simulink model "SimulinkModelMatlab2022bStudents"  (R2025b)
settings: Solver=VariableStepAuto  StartTime=0.0  StopTime=5e-5  RelTol=1e-3
values from neighbouring files (symbols this model uses):
  Ad = sysDiscreteZOH.A    [pt1.m]
  Bd = sysDiscreteZOH.B    [pt1.m]
  Cd = sysDiscreteZOH.C    [pt1.m]
  Rnsim = 0.0025    [pt1.m]
  Rvsim = [0.025 0; 0 1e-6]    [pt1.m]
  Ts = 2*pi / (10* wn)    [Kalman_code.m]    (also in pt1.m = 2.5e-07)
settings Model: Creator=Freja  LastModifiedBy=Lenovo
settings DataIOCC: ReturnWorkspaceOutputs=off
settings OptimizationCC: ReuseModelBlockBuffer=off
settings RTWCC: GPUComputeCapability=3.5

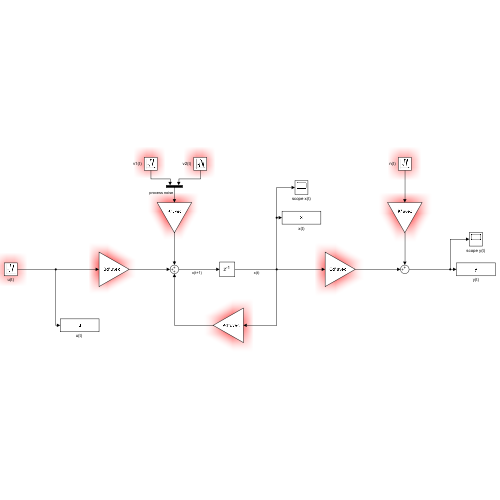
[thumbnail: Simulink's stored preview of the top-level diagram]
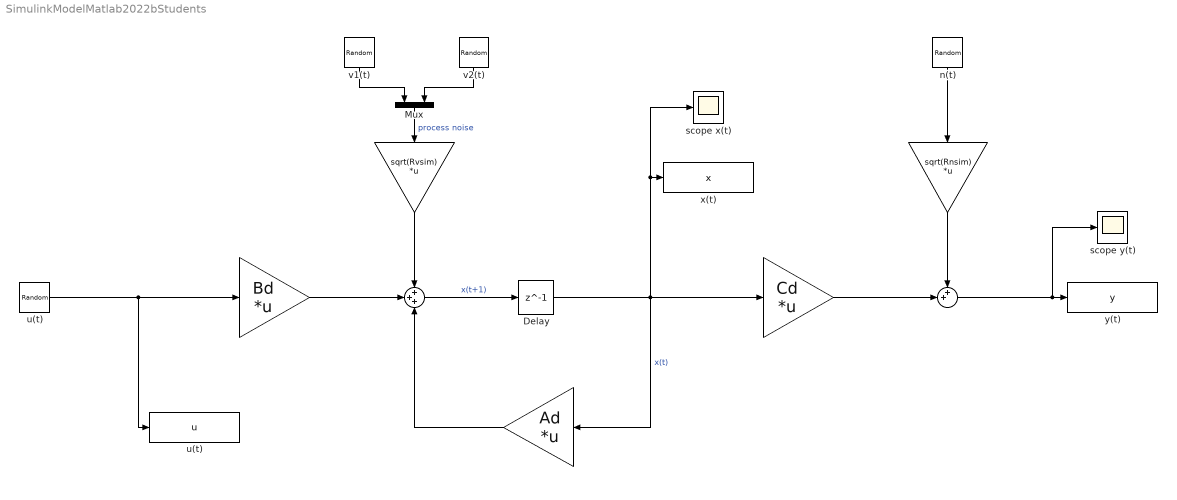
== system SimulinkModelMatlab2022bStudents ==
  " " : Gain  Gain=Bd  Multiplication=Matrix(K*u) (u vector)
  "  " : Sum  Inputs=+++
  "   " : Gain  Gain=Cd  Multiplication=Matrix(K*u) (u vector)
  "     " : Gain  Gain=Ad  Multiplication=Matrix(K*u) (u vector)
  "        " : Sum  Inputs=++|
  "         " : Gain  Gain=sqrt(Rvsim)  Multiplication=Matrix(K*u) (u vector)
  "                " : Gain  Gain=sqrt(Rnsim)  Multiplication=Matrix(K*u) (u vector)
  Delay : Delay  DelayLength=1
  Mux : Mux  Inputs=2
  n(t) : RandomNumber  SampleTime=Ts
  scope x(t) : Scope
      settings: ActiveDisplayYMinimum=-0.40895  ActiveDisplayYMaximum=0.5797
  scope y(t) : Scope
      settings: ActiveDisplayYMinimum=-0.40246  ActiveDisplayYMaximum=0.57208
  u(t) : RandomNumber  SampleTime=Ts
  "u(t) " : ToWorkspace  VariableName=u  SaveFormat=Timeseries  SampleTime=-1
  v1(t) : RandomNumber  SampleTime=Ts
  v2(t) : RandomNumber  SampleTime=Ts
  x(t) : ToWorkspace  VariableName=x  SaveFormat=Timeseries  SampleTime=-1
  y(t) : ToWorkspace  VariableName=y  SaveFormat=Timeseries  SampleTime=-1
  wires:
  Delay/1 -> "     "/1, scope x(t)/1, x(t)/1, "   "/1  "x(t)"
  "   "/1 -> "        "/2
  "        "/1 -> scope y(t)/1, y(t)/1
  "  "/1 -> Delay/1  "x(t+1)"
  "     "/1 -> "  "/3
  " "/1 -> "  "/2
  u(t)/1 -> "u(t) "/1, " "/1
  "         "/1 -> "  "/1
  "                "/1 -> "        "/1
  n(t)/1 -> "                "/1
  v2(t)/1 -> Mux/2
  Mux/1 -> "         "/1  "process noise"
  v1(t)/1 -> Mux/1
